simulink model "integrator_reset"  (R2022a)
settings: Solver=FixedStepAuto  StartTime=0.0  StopTime=20  FixedStep=0.1  RelTol=1e-3
libraries: simulink x2
settings Model: SnapshotInterval=1  Creator=Stefano Paracchino  LastModifiedBy=Stefano Paracchino

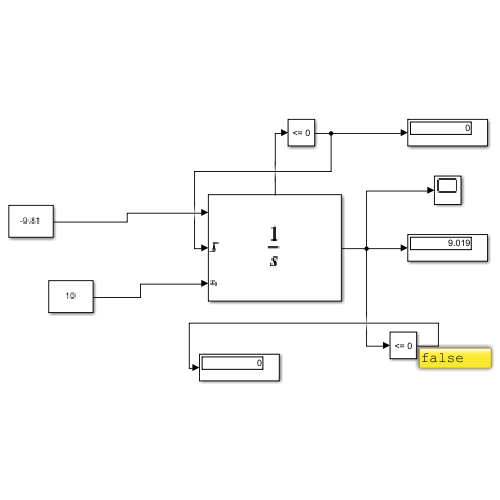
[thumbnail: Simulink's stored preview of the top-level diagram]
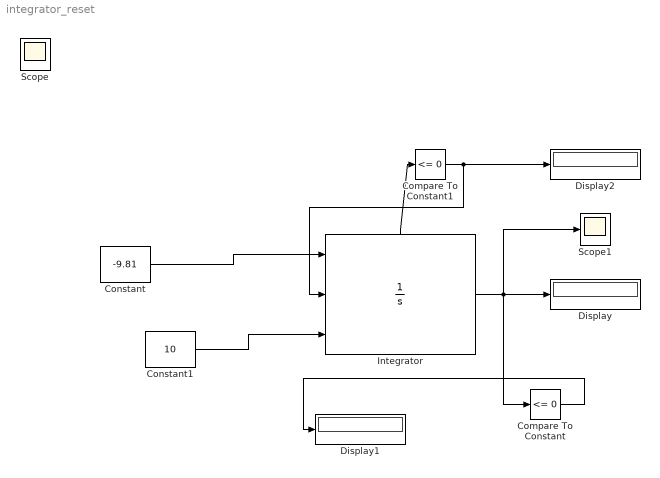
== system integrator_reset ==
  Compare To Constant : simulink/Logic and Bit Operations/Compare To Constant  relop=<=  const=0  OutDataTypeStr=boolean
  Compare To Constant1 : simulink/Logic and Bit Operations/Compare To Constant  relop=<=  const=0  OutDataTypeStr=boolean
  Constant : Constant  Value=-9.81
  Constant1 : Constant  Value=10
  Display : Display
  Display1 : Display
  Display2 : Display
  Integrator : Integrator  ExternalReset=rising  InitialConditionSource=external  ShowStatePort=on
  Scope1 : Scope
  Scope : Scope
  wires:
  Constant/1 -> Integrator/1
  Integrator/1 -> Display/1, Scope1/1, Compare To Constant/1
  Compare To Constant/1 -> Display1/1
  Constant1/1 -> Integrator/3
  Integrator/State -> Compare To Constant1/1
  Compare To Constant1/1 -> Integrator/2, Display2/1
